simulink model "MotorXploer"  (R2024b)
settings: Solver=FixedStepAuto  StartTime=0.0  StopTime=inf  FixedStep=0.001  RelTol=1e-3  EnableMultiTasking=on
values from neighbouring files (symbols this model uses):
  n = ((-(maxSpeed/stallTorque)*((Torque1).^2) + maxSpeed*Torque1) ./      (((I_Stall - I_No_load)/stallTorque)*Torque1*Vin + I_No_load*Vin)) * 100    [UnitedPlot.m]
undefined symbols (not defined in the file or in its folder): Blocking, LF, Non
libraries: hdlsllib x5, amg_usbconverter_n_connect_lib x3, simulink x1
settings Model: Creator=beamk  LastModifiedBy=Lenovo
settings OptimizationCC: DefaultParameterBehavior=Inlined  EnhancedBackFolding=on  PassReuseOutputArgsAs=Individual arguments  ZeroExternalMemoryAtStartup=off  ZeroInternalMemoryAtStartup=off  MaxStackSize=512  OptimizeBlockOrder=speed  DifferentSizesBufferReuse=on  OptimizationCustomize=off  EfficientTunableParamExpr=on
settings DebuggingCC: ParameterTunabilityLossMsg=error
settings HardwareCC: ProdBitPerPointer=32  ProdBitPerSizeT=32  ProdBitPerPtrDiffT=32  ProdLargestAtomicInteger=Long  ProdLargestAtomicFloat=Double  ProdWordSize=32  ProdLongLongMode=on  ProdHWDeviceType=ARM Compatible->ARM Cortex-M
settings SFSimCC: MATLABDynamicMemAlloc=off
settings RTWCC: Description=Embedded Coder  SystemTargetFile=ert.tlc  HardwareBoard=STM32G4xx Based  TemplateMakefile=ert_default_tmf  Toolchain=GNU Tools for ARM Embedded Processors
settings CodeAppCC: ForceParamTrailComments=on  IgnoreCustomStorageClasses=off  OperatorAnnotations=on  SimulinkDataObjDesc=on  SFDataObjDesc=on  InsertBlockDesc=on
settings ERTTargetCC: TargetLangStandard=C99 (ISO)  CodeReplacementLibrary=ARM Cortex-M  ExtModeTransport=3  ExtModeStaticAlloc=on  ExtModeStaticAllocSize=2048  ExtModeMexFile=ext_xcp  ExtModeIntrfLevel=Level2 - Open

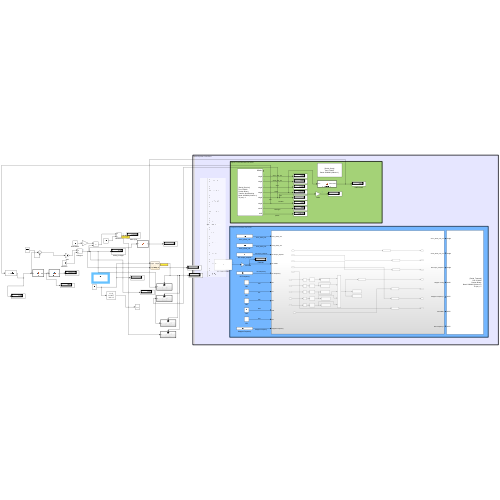
[thumbnail: Simulink's stored preview of the top-level diagram]
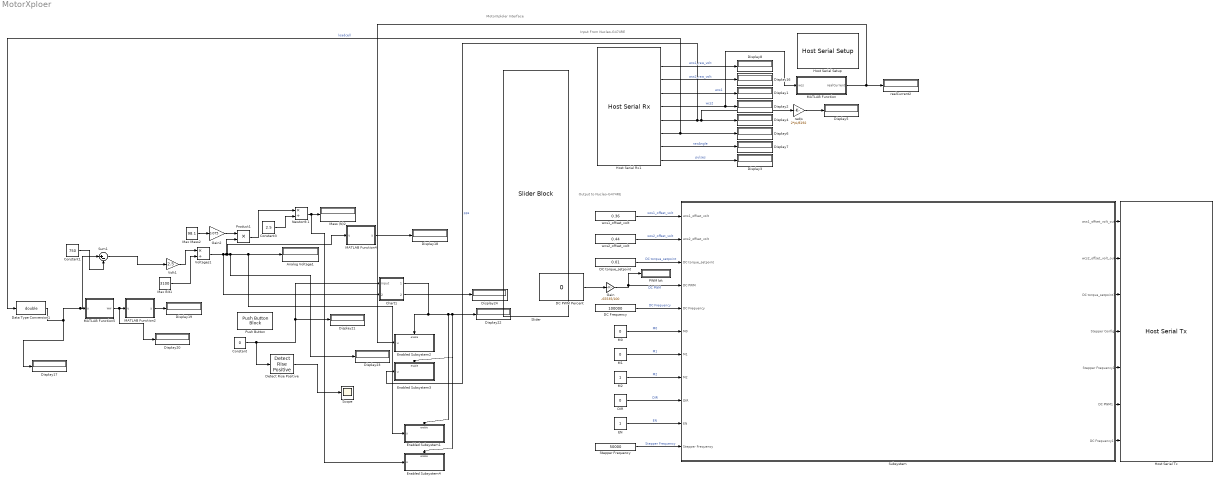
== system MotorXploer ==
  note: Output to Nucleo-G474RE
  note: Input From Nucleo-G474RE
  note: MotorXploler Interface
  Analog Voltage1 : Display
  Chart1 : Stateflow chart  TreatAsAtomicUnit=on
  Constant : Constant  Value=0
  Constant1 : Constant  Value=750
  Constant3 : Constant  Value=2.5
  DC Frequency : Constant  Value=100000
  DC PWM Percent : Constant  Value=0
  DC torque_setpoint : Constant  Value=0.01
  DIR : Constant  Value=0  OutDataTypeStr=uint8
  Data Type Conversion1 : DataTypeConversion  OutDataTypeStr=double  SaturateOnIntegerOverflow=off  RndMeth=Floor
  Detect Rise Positive : simulink/Logic and Bit Operations/Detect Rise Positive  vinit=0  OutDataTypeStr=boolean
  Display{1..8,16..24} (17 alike) : Display
      Display19 settings: Format=short_e
  EN : Constant  OutDataTypeStr=uint8
  Enabled Subsystem1 : Subsystem  TreatAsAtomicUnit=on
  Enabled Subsystem2 : Subsystem  TreatAsAtomicUnit=on
  Enabled Subsystem3 : Subsystem  TreatAsAtomicUnit=on
  Enabled Subsystem4 : Subsystem  TreatAsAtomicUnit=on
  Gain : Gain  Gain=-65535/100
  Gain2 : Gain  Gain=0.075
  Host Serial Rx1 : amg_usbconverter_n_connect_lib/Host Serial Rx  conf=rx  port=<auto>  baudrate=2000000  databits=8  parity=None  stopbit=1  flowcontrol=None  transfer=Non-Blocking  timeout=5  packetmode=Binary  enableinitialvalues=off  initialvalues=[]  binheader='45'  binterminator='A'  porttype_double=0  porttype_single=6  porttype_int8=0  porttype_uint8=0  porttype_int16=0  porttype_uint16=1  porttype_int32=1  porttype_uint32=0  asciiformat='%f,%f,%d,%d'  rx_asciiterminator="LF (0x0A - \"\\n\")"  tx_asciiterminator="CRLF (0x0D 0x0A - \"\\r\\n\")"  sampletime=-1  enablecustomportlabel=off  cinputportlabel=0  coutputportlabel=A  portpinstr=0  blockid=HostSerialRx1  inputporttype=[]  inputportwidth=[]  inputportlabel={}  outputporttype=[3 1 1 1 1 1 1 5 6]  outputportwidth=[1 1 1 1 1 1 1 1 1]  outputportlabel={'READY','single','single','single','single','single','single','uint16','int32'}  compat=0  optionstring=[]  autoport='COM12'
  Host Serial Setup : amg_usbconverter_n_connect_lib/Host Serial Setup  conf=setup  port=<auto>  baudrate=2000000  databits=8  parity=None  stopbit=1  flowcontrol=None  transfer=Blocking  timeout=2  packetmode=Binary  initialvalues=[]  binheader='7E 7E'  binterminator='03 03'  porttype_double=0  porttype_single=1  porttype_int8=0  porttype_uint8=0  porttype_int16=0  porttype_uint16=0  porttype_int32=0  porttype_uint32=2  asciiformat='%d %u %x'  rx_asciiterminator="CRLF (0x0D 0x0A - \"\\r\\n\")"  tx_asciiterminator="CRLF (0x0D 0x0A - \"\\r\\n\")"  sampletime=-1  enablecustomportlabel=off  cinputportlabel=0  coutputportlabel=A  portpinstr=0  blockid=HostSerialSetup  inputporttype=[]  inputportwidth=[]  inputportlabel={}  outputporttype=[]  outputportwidth=[]  outputportlabel={}  compat=0  optionstring=[]  autoport='COM12'
  Host Serial Tx : amg_usbconverter_n_connect_lib/Host Serial Tx  conf=tx  port=<auto>  baudrate=2000000  databits=8  parity=None  stopbit=1  flowcontrol=None  transfer=Blocking  timeout=2  packetmode=Binary  initialvalues=[]  binheader='45'  binterminator='A'  porttype_double=0  porttype_single=3  porttype_int8=0  porttype_uint8=1  porttype_int16=0  porttype_uint16=0  porttype_int32=3  porttype_uint32=0  asciiformat='%d,%f'  rx_asciiterminator="CRLF (0x0D 0x0A - \"\\r\\n\")"  tx_asciiterminator="CRLF (0x0D 0x0A - \"\\r\\n\")"  sampletime=-1  enablecustomportlabel=off  cinputportlabel=0  coutputportlabel=A  portpinstr=0  blockid=HostSerialTx  inputporttype=[1 1 1 3 6 6 6]  inputportwidth=[1 1 1 1 1 1 1]  inputportlabel={'single','single','single','uint8','int32','int32','int32'}  outputporttype=[]  outputportwidth=[]  outputportlabel={}  compat=0  optionstring=[]  autoport='COM12'
      settings: SourceProductName=aMG USB Converter N
  M0 : Constant  Value=0  OutDataTypeStr=uint8
  M1 : Constant  Value=0  OutDataTypeStr=uint8
  M2 : Constant  OutDataTypeStr=uint8
  MATLAB Function : MATLAB Function  TreatAsAtomicUnit=on
  MATLAB Function2 : MATLAB Function  TreatAsAtomicUnit=on
  MATLAB Function4 : MATLAB Function  TreatAsAtomicUnit=on
  MATLAB Function5 : MATLAB Function  TreatAsAtomicUnit=on
  Mass (N)2 : Display
  Max Bit1 : Constant  Value=3100
  Max Mass2 : Constant  Value=98.1
  Newton9.1 : Product  Inputs=*/
  PWM bit : Display
  Product1 : Product
  Push Button : PushButtonBlock  OffValue=0.000000
  Scope : Scope
  Slider : SliderBlock  ScaleMin=-65535  ScaleMax=65535
  Stepper Frequency : Constant  Value=50000
  Subsystem : Subsystem
  Sum1 : Sum  Inputs=|+-
  Volt1 : Gain  Gain=2.5
  Voltages1 : Product  Inputs=*/
  rad/s : Gain  Gain=2*pi/8192
  realCurrent2 : Display
  wcs1_offset_volt : Constant  Value=0.36  OutDataTypeStr=single
  wcs2_offset_volt : Constant  Value=0.44  OutDataTypeStr=single
  wires:
  Host Serial Rx1/2 -> Display8/1  "wcs1_raw_volt"
  Host Serial Rx1/3 -> Display16/1  "wcs2_raw_volt"
  Host Serial Rx1/7 -> Data Type Conversion1/1, Display6/1  "loadcell"
  Host Serial Rx1/5 -> MATLAB Function/1(wcs), Display2/1  "wcs2"
  Host Serial Rx1/8 -> Display7/1  "rawAngle"
  rad/s/1 -> Display5/1
  Host Serial Rx1/6 -> Enabled Subsystem3/1(u), Display4/1, rad/s/1  "pps"
  Host Serial Rx1/4 -> Display1/1  "wcs1"
  Host Serial Rx1/9 -> Display3/1  "pulses"
  wcs1_offset_volt/1 -> Subsystem/1(wcs1_offset_volt)  "wcs1_offset_volt"
  wcs2_offset_volt/1 -> Subsystem/2(wcs2_offset_volt)  "wcs2_offset_volt"
  DC torque_setpoint/1 -> Subsystem/3(DC torque_setpoint)  "DC torque_setpoint"
  DC Frequency/1 -> Subsystem/5(DC Frequency)  "DC Frequency"
  M0/1 -> Subsystem/6(M0)  "M0"
  M1/1 -> Subsystem/7(M1)  "M1"
  M2/1 -> Subsystem/8(M2)  "M2"
  DIR/1 -> Subsystem/9(DIR)  "DIR"
  EN/1 -> Subsystem/10(EN)  "EN"
  Stepper Frequency/1 -> Subsystem/11(Stepper Frequency)  "Stepper Frequency"
  Subsystem/1(wcs1_offset_volt_out) -> Host Serial Tx/1
  Subsystem/2(wcs2_offset_volt_out) -> Host Serial Tx/2
  Subsystem/3(DC torque_setpoint1) -> Host Serial Tx/3
  Subsystem/4(Stepper Config) -> Host Serial Tx/4
  Subsystem/5(Stepper Frequency1) -> Host Serial Tx/5
  Subsystem/6(DC PWM1) -> Host Serial Tx/6
  Subsystem/7(DC Frequency1) -> Host Serial Tx/7
  Gain2/1 -> Product1/1
  Constant1/1 -> Sum1/2
  Sum1/1 -> Volt1/1
  Max Mass2/1 -> Gain2/1
  Constant3/1 -> Newton9.1/2
  MATLAB Function2/1(y) -> Display19/1
  Volt1/1 -> Voltages1/1
  MATLAB Function4/1(y) -> Display18/1
  Max Bit1/1 -> Voltages1/2
  Chart1/2(time_dis) -> Display24/1
  Data Type Conversion1/1 -> Sum1/1, MATLAB Function5/1(u), Display17/1
  Constant/1 -> Detect Rise Positive/1, Chart1/1(input), Display21/1
  MATLAB Function5/1(ww) -> Display20/1, MATLAB Function2/1(u)
  Product1/1 -> Newton9.1/1
  Detect Rise Positive/1 -> Scope/1
  DC PWM Percent/1 -> Gain/1
  Gain/1 -> Subsystem/4(DC PWM), PWM bit/1  "DC PWM"
  MATLAB Function/1(realCurrent) -> Enabled Subsystem2/1(u), realCurrent2/1
  Voltages1/1 -> Chart1/2(outputvolt), Product1/2, MATLAB Function4/1(u), Enabled Subsystem1/1(u), Analog Voltage1/1, Display23/1
  Chart1/1(output) -> Display22/1, Enabled Subsystem4/Enable, Enabled Subsystem3/Enable, Enabled Subsystem1/Enable, Enabled Subsystem2/Enable
  Newton9.1/1 -> Enabled Subsystem4/1(u), Mass (N)2/1

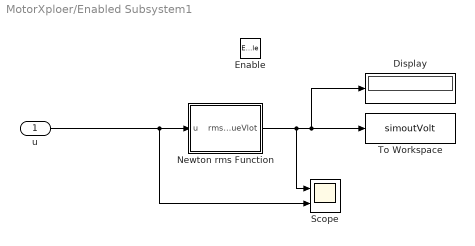
== system MotorXploer/Enabled Subsystem1 ==
  u : Inport
  Enable : EnablePort
  Display : Display
  Newton rms Function : MATLAB Function  TreatAsAtomicUnit=on
  Scope : Scope  NumInputPorts=2
  To Workspace : ToWorkspace  VariableName=simoutVolt  SaveFormat=Timeseries  SampleTime=-1
  wires:
  u/1 -> Scope/2, Newton rms Function/1(u)
  Newton rms Function/1(rms_valueVlot) -> Scope/1, Display/1, To Workspace/1

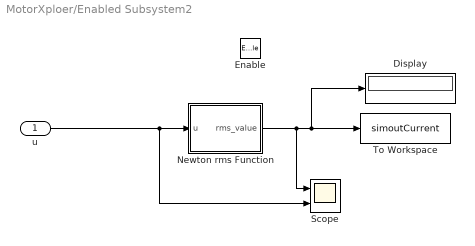
== system MotorXploer/Enabled Subsystem2 ==
  u : Inport
  Enable : EnablePort
  Display : Display
  Newton rms Function : MATLAB Function  TreatAsAtomicUnit=on
  Scope : Scope  NumInputPorts=2
  To Workspace : ToWorkspace  VariableName=simoutCurrent  SaveFormat=Timeseries  SampleTime=-1
  wires:
  u/1 -> Scope/2, Newton rms Function/1(u)
  Newton rms Function/1(rms_value) -> Scope/1, Display/1, To Workspace/1

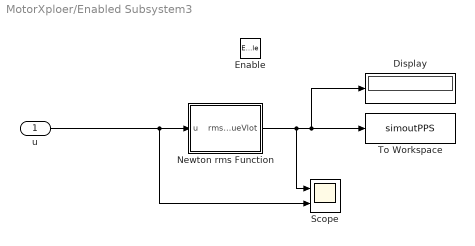
== system MotorXploer/Enabled Subsystem3 ==
  u : Inport
  Enable : EnablePort
  Display : Display
  Newton rms Function : MATLAB Function  TreatAsAtomicUnit=on
  Scope : Scope  NumInputPorts=2
  To Workspace : ToWorkspace  VariableName=simoutPPS  SaveFormat=Timeseries  SampleTime=-1
  wires:
  u/1 -> Scope/2, Newton rms Function/1(u)
  Newton rms Function/1(rms_valueVlot) -> Scope/1, Display/1, To Workspace/1

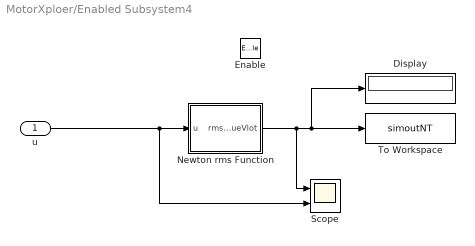
== system MotorXploer/Enabled Subsystem4 ==
  u : Inport
  Enable : EnablePort
  Display : Display
  Newton rms Function : MATLAB Function  TreatAsAtomicUnit=on
  Scope : Scope  NumInputPorts=2
  To Workspace : ToWorkspace  VariableName=simoutNT  SaveFormat=Timeseries  SampleTime=-1
  wires:
  u/1 -> Scope/2, Newton rms Function/1(u)
  Newton rms Function/1(rms_valueVlot) -> Scope/1, Display/1, To Workspace/1

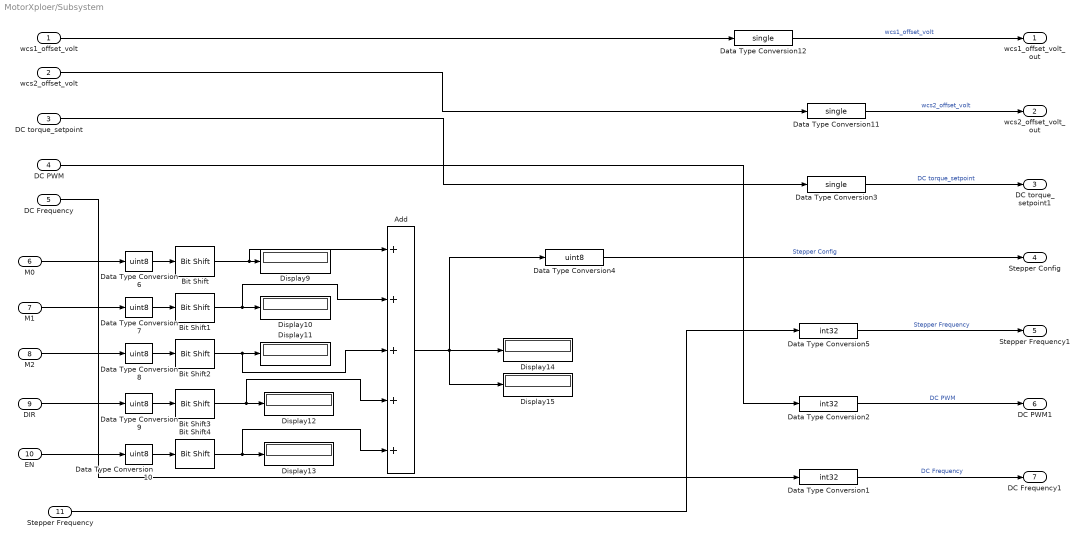
== system MotorXploer/Subsystem ==
  wcs1_offset_volt : Inport
  wcs2_offset_volt : Inport  Port=2
  DC torque_setpoint : Inport  Port=3
  DC PWM : Inport  Port=4
  DC Frequency : Inport  Port=5
  M0 : Inport  Port=6
  M1 : Inport  Port=7
  M2 : Inport  Port=8
  DIR : Inport  Port=9
  EN : Inport  Port=10
  Stepper Frequency : Inport  Port=11
  Add : Sum  Inputs=+++++
  Bit Shift : hdlsllib/Logic and Bit Operations/Bit Shift  mode=Shift Left Logical  N=4
  Bit Shift1 : hdlsllib/Logic and Bit Operations/Bit Shift  mode=Shift Left Logical  N=3
  Bit Shift2 : hdlsllib/Logic and Bit Operations/Bit Shift  mode=Shift Left Logical  N=2
  Bit Shift3 : hdlsllib/Logic and Bit Operations/Bit Shift  mode=Shift Left Logical  N=1
  Bit Shift4 : hdlsllib/Logic and Bit Operations/Bit Shift  mode=Shift Left Logical  N=0
  Data Type Conversion1 : DataTypeConversion  OutDataTypeStr=int32  SaturateOnIntegerOverflow=off  RndMeth=Floor
  Data Type Conversion{4,6..10} (6 alike) : DataTypeConversion  OutDataTypeStr=uint8  SaturateOnIntegerOverflow=off  RndMeth=Floor
  Data Type Conversion11 : DataTypeConversion  OutDataTypeStr=single  SaturateOnIntegerOverflow=off  RndMeth=Floor
  Data Type Conversion12 : DataTypeConversion  OutDataTypeStr=single  SaturateOnIntegerOverflow=off  RndMeth=Floor
  Data Type Conversion2 : DataTypeConversion  OutDataTypeStr=int32  SaturateOnIntegerOverflow=off  RndMeth=Floor
  Data Type Conversion3 : DataTypeConversion  OutDataTypeStr=single  SaturateOnIntegerOverflow=off  RndMeth=Floor
  Data Type Conversion5 : DataTypeConversion  OutDataTypeStr=int32  SaturateOnIntegerOverflow=off  RndMeth=Floor
  Display{9..15} (7 alike) : Display
      Display10 settings: Format=binary (Stored Integer)
      Display11 settings: Format=binary (Stored Integer)
      Display12 settings: Format=binary (Stored Integer)
      Display13 settings: Format=binary (Stored Integer)
      Display14 settings: Format=binary (Stored Integer)
      Display9 settings: Format=binary (Stored Integer)
  wcs1_offset_volt_out : Outport
  wcs2_offset_volt_out : Outport  Port=2
  DC torque_setpoint1 : Outport  Port=3
  Stepper Config : Outport  Port=4
  Stepper Frequency1 : Outport  Port=5
  DC PWM1 : Outport  Port=6
  DC Frequency1 : Outport  Port=7
  wires:
  Bit Shift/1 -> Display9/1, Add/1
  Data Type Conversion8/1 -> Bit Shift2/1
  EN/1 -> Data Type Conversion10/1
  Data Type Conversion6/1 -> Bit Shift/1
  DC torque_setpoint/1 -> Data Type Conversion3/1
  Data Type Conversion2/1 -> DC PWM1/1  "DC PWM"
  Data Type Conversion7/1 -> Bit Shift1/1
  Data Type Conversion10/1 -> Bit Shift4/1
  DC PWM/1 -> Data Type Conversion2/1
  Bit Shift3/1 -> Display12/1, Add/4
  Data Type Conversion12/1 -> wcs1_offset_volt_out/1  "wcs1_offset_volt"
  Add/1 -> Display15/1, Display14/1, Data Type Conversion4/1
  Bit Shift2/1 -> Display11/1, Add/3
  Stepper Frequency/1 -> Data Type Conversion5/1
  M1/1 -> Data Type Conversion7/1
  Bit Shift1/1 -> Display10/1, Add/2
  Bit Shift4/1 -> Display13/1, Add/5
  M0/1 -> Data Type Conversion6/1
  Data Type Conversion9/1 -> Bit Shift3/1
  Data Type Conversion11/1 -> wcs2_offset_volt_out/1  "wcs2_offset_volt"
  M2/1 -> Data Type Conversion8/1
  wcs1_offset_volt/1 -> Data Type Conversion12/1
  DC Frequency/1 -> Data Type Conversion1/1
  wcs2_offset_volt/1 -> Data Type Conversion11/1
  Data Type Conversion1/1 -> DC Frequency1/1  "DC Frequency"
  DIR/1 -> Data Type Conversion9/1
  Data Type Conversion4/1 -> Stepper Config/1  "Stepper Config"
  Data Type Conversion3/1 -> DC torque_setpoint1/1  "DC torque_setpoint"
  Data Type Conversion5/1 -> Stepper Frequency1/1  "Stepper Frequency"

== matlab function MotorXploer/Enabled Subsystem1/Newton rms Function ==
  data: u input; rms_valueVlot output
function rms_valueVlot = fcn(u)
    % Get the size of input data u
    n = 1;  % Determine how many elements are in u
    
    % Initialize an array to store the 1000 data points
    persistent data_array;  % Use persistent to store data across function calls
    persistent count;       % To keep track of how many data points have been stored
    
    if isempty(data_array)
        data_array = zeros(1000, 1);  % Preallocate space for 1000 data points
        count = 0;                    % Initialize the count
    end
    
    % Loop through each element of the input data and store it
    for i = 1:n
        if count < 1000
            count = count + 1;
            data_array(count) = u(i);  % Store the data
        end
    end
    
    % Once 1000 data points have been stored, calculate the RMS
    if count == 1000
        % Calculate the RMS value
        rms_valueVlot = sqrt(mean(data_array.^2));
        
        % Reset the count and data_array if needed for continuous calculations
        count = 0;
        data_array = zeros(1000, 1);
    else
        rms_valueVlot = NaN;  % Output NaN until 1000 points have been collected
    end
   
end

== matlab function MotorXploer/MATLAB Function ==
  data: wcs input; realCurrent output
function realCurrent = toRealCurrent(wcs)


realCurrent = 20.56*(wcs^2) + 2053.23*wcs -145.70;

== matlab function MotorXploer/Enabled Subsystem4/Newton rms Function ==
  data: u input; rms_valueVlot output
function rms_valueVlot = fcn(u)
    % Get the size of input data u
    n = 1;  % Determine how many elements are in u
    
    % Initialize an array to store the 1000 data points
    persistent data_array;  % Use persistent to store data across function calls
    persistent count;       % To keep track of how many data points have been stored
    
    if isempty(data_array)
        data_array = zeros(1000, 1);  % Preallocate space for 1000 data points
        count = 0;                    % Initialize the count
    end
    
    % Loop through each element of the input data and store it
    for i = 1:n
        if count < 1000
            count = count + 1;
            data_array(count) = u(i);  % Store the data
        end
    end
    
    % Once 1000 data points have been stored, calculate the RMS
    if count == 1000
        % Calculate the RMS value
        rms_valueVlot = sqrt(mean(data_array.^2));
        
        % Reset the count and data_array if needed for continuous calculations
        count = 0;
        data_array = zeros(1000, 1);
    else
        rms_valueVlot = NaN;  % Output NaN until 1000 points have been collected
    end
   
end

== stateflow chart MotorXploer/Chart1 ==
  state initial
    entry:
    time=0;
    outputvolt;
    output= 0;
  state State
    entry:
    output = 1;
    during:
    time = time + 0.001;
    time_dis = time;
    exit:
    output = 0;
    time = 0;
  (default) -> initial
  initial -> State : [input == 1]
  State -> initial : [time >= 1]
  data: input input; outputvolt input; output output; time local; time_dis output

== matlab function MotorXploer/Enabled Subsystem2/Newton rms Function ==
  data: u input; rms_value output
function rms_value = fcn(u)
    % Get the size of input data u
    n = 1;  % Determine how many elements are in u
    
    % Initialize an array to store the 1000 data points
    persistent data_array;  % Use persistent to store data across function calls
    persistent count;       % To keep track of how many data points have been stored
    
    if isempty(data_array)
        data_array = zeros(1000, 1);  % Preallocate space for 1000 data points
        count = 0;                    % Initialize the count
    end
    
    % Loop through each element of the input data and store it
    for i = 1:n
        if count < 1000
            count = count + 1;
            data_array(count) = u(i);  % Store the data
        end
    end
    
    % Once 1000 data points have been stored, calculate the RMS
    if count == 1000
        % Calculate the RMS value
        rms_value = sqrt(mean(data_array.^2));
        
        % Reset the count and data_array if needed for continuous calculations
        count = 0;
        data_array = zeros(1000, 1);
    else
        rms_value = NaN;  % Output NaN until 1000 points have been collected
    end
   
end

== matlab function MotorXploer/Enabled Subsystem3/Newton rms Function ==
  data: u input; rms_valueVlot output
function rms_valueVlot = fcn(u)
    % Get the size of input data u
    n = 1;  % Determine how many elements are in u
    
    % Initialize an array to store the 1000 data points
    persistent data_array;  % Use persistent to store data across function calls
    persistent count;       % To keep track of how many data points have been stored
    
    if isempty(data_array)
        data_array = zeros(1000, 1);  % Preallocate space for 1000 data points
        count = 0;                    % Initialize the count
    end
    
    % Loop through each element of the input data and store it
    for i = 1:n
        if count < 1000
            count = count + 1;
            data_array(count) = u(i);  % Store the data
        end
    end
    
    % Once 1000 data points have been stored, calculate the RMS
    if count == 1000
        % Calculate the RMS value
        rms_valueVlot = sqrt(mean(data_array.^2));
        
        % Reset the count and data_array if needed for continuous calculations
        count = 0;
        data_array = zeros(1000, 1);
    else
        rms_valueVlot = NaN;  % Output NaN until 1000 points have been collected
    end
   
end

== matlab function MotorXploer/MATLAB Function2 ==
  data: u input; y output
function y = fcn(u)
y = u/0.3;
if y <0
    y=0;
end

== matlab function MotorXploer/MATLAB Function4 ==
  data: u input; y output
function y = fcn(u)
y = u/0.31;
if y <0
    y=0;
end

== matlab function MotorXploer/MATLAB Function5 ==
  data: u input; ww output
function ww= fcn(u)
ww = u -30;
if(ww < 0)
    ww = 0;
end
